simulink model "Mark60"  (Simulink 10.0)
settings: Solver=FixedStepAuto  StartTime=0.0  StopTime=4000  FixedStep=0.01  RelTol=1e-3  EnableMultiTasking=on
values from neighbouring files (symbols this model uses):
  A = 2.2    [constant（final）.m]
  c = 10800*0.9    (= 9720)    [constant（final）.m]
  C_D = 0.35    [constant（final）.m]
  C_e = 4.4    [constant（final）.m]
  C_t = 42    [constant（final）.m]
  Cb = interp1(SOC0,Cb0,SOC, 'spline')    [constant（final）.m]
  f = 0.018    [constant（final）.m]
  g = 9.8    [constant（final）.m]
  i_g = 2    [constant（final）.m]
  J_m = 0.25    [constant（final）.m]
  J_w = 4    [constant（final）.m]
  K_p = 4    [constant（final）.m]
  m = 1000    [constant（final）.m]
  Phi = 0.028    [constant（final）.m]
  r_w = 0.28    [constant（final）.m]
  Ra = 0.088    [constant（final）.m]
  Ro = interp1(SOC0,Ro0,SOC, 'spline')    [constant（final）.m]
  rou = 1.226    [constant（final）.m]
  Rp = interp1(SOC0,Rp0,SOC, 'spline')    [constant（final）.m]
  SOC = 0:0.0001:1    [constant（final）.m]
  T_i = 1    [constant（final）.m]
  tao = interp1(SOC0,tao0,SOC, 'spline')    [constant（final）.m]
  Uoc = UUoc*4.2/UUoc(10001)    [constant（final）.m]
  yita = 0.8    [constant（final）.m]
libraries: SignalEditorBlockLib x1
settings Model: Creator=TonyStark  LastModifiedBy=TonyStark
settings SolverCC: AutoInsertRateTranBlk=on
settings DataIOCC: LimitDataPoints=on  SignalLoggingSaveFormat=ModelDataLogs
settings OptimizationCC: ExpressionDepthLimit=2147483647
settings DebuggingCC: SolverPrmCheckMsg=warning  FcnCallInpInsideContextMsg=warning  StateNameClashWarn=warning
settings GRTTargetCC: GeneratePreprocessorConditionals=Disable all
settings ConfigComp: CovExternalEMLEnable=off

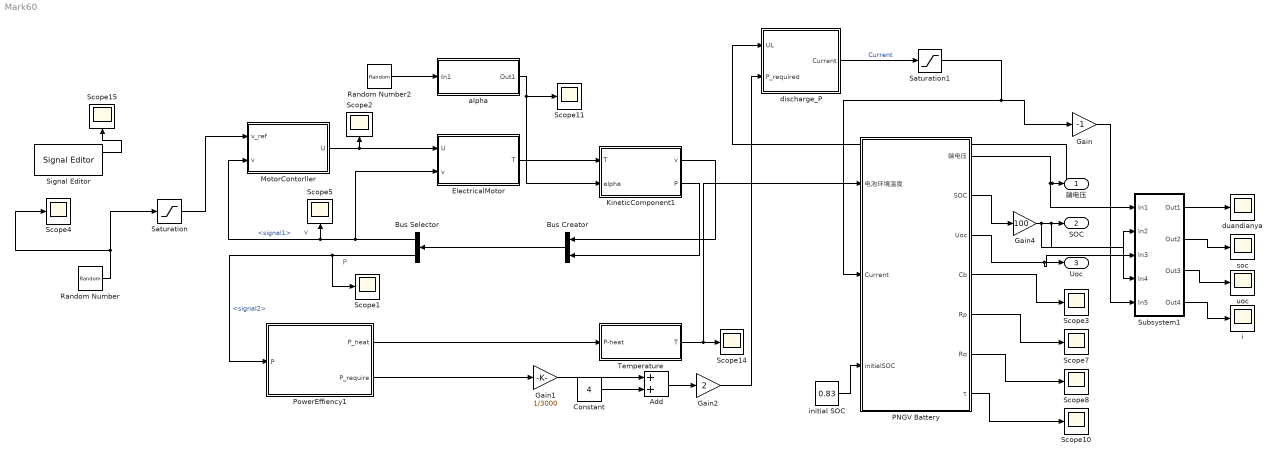
== system Mark60 ==
  note: v
  note: P
  Add : Sum
  Bus Creator : BusCreator  Inputs=2
  Bus Selector : BusSelector  OutputSignals=signal1,signal2
  Constant : Constant  Value=4
  ElectricalMotor : Subsystem
  Gain : Gain  Gain=-1
  Gain1 : Gain  Gain=1/3000
  Gain2 : Gain  Gain=2
  Gain4 : Gain  Gain=100
  KineticComponent1 : Subsystem
  MotorContorller : Subsystem
  PNGV Battery : Subsystem
  PowerEffiency1 : Subsystem
  Random Number : RandomNumber  Mean=13  Variance=2.5  Seed=2  SampleTime=0.01
  Random Number2 : RandomNumber  SampleTime=1
  Saturation : Saturate  UpperLimit=30  LowerLimit=0
  Saturation1 : Saturate  UpperLimit=100  LowerLimit=-100
  Scope{1..5,7..8,10..11,14..15} (11 alike) : Scope
  Signal Editor : SignalEditorBlockLib/Signal Editor  FileName=t1.mat  ActiveScenario=Scenario  ActiveSignal=Signal1  IsBus=off  OutputBusObjectStr=Bus: BusObject  SampleTime=0  Interpolate=off  ZeroCross=off  OutputAfterFinalValue=Setting to zero  Unit=inherit  PreserveSignalName=on
      settings: SourceProductName=Simulink
  Subsystem1 : Subsystem
  Temperature : Subsystem
  alpha : Subsystem
  discharge_P : Subsystem
  duandianya : Scope
  "i " : Scope
  initial SOC : Constant  Value=0.83
  "soc " : Scope
  "uoc " : Scope
  端电压 : Outport  VectorParamsAs1DForOutWhenUnconnected=off
  SOC : Outport  Port=2  VectorParamsAs1DForOutWhenUnconnected=off
  Uoc : Outport  Port=3  VectorParamsAs1DForOutWhenUnconnected=off
  wires:
  MotorContorller/1(U) -> ElectricalMotor/1(U), Scope2/1
  Bus Creator/1 -> Bus Selector/1
  Bus Selector/1 -> Scope5/1, MotorContorller/2(v), ElectricalMotor/2(v)  "<signal1>"
  KineticComponent1/1(v) -> Bus Creator/1
  KineticComponent1/2(P) -> Bus Creator/2
  ElectricalMotor/1(T) -> KineticComponent1/1(T)
  Bus Selector/2 -> Scope1/1, PowerEffiency1/1(P)  "<signal2>"
  PowerEffiency1/1(P_heat) -> Temperature/1(P-heat)
  Random Number2/1 -> alpha/1(In1)
  alpha/1(Out1) -> KineticComponent1/2(alpha), Scope11/1
  PNGV Battery/6(Ro) -> Scope8/1
  discharge_P/1(Current) -> Saturation1/1  "Current"
  Temperature/1(T) -> PNGV Battery/1(电池环境温度), Scope14/1
  Gain4/1 -> Subsystem1/4(In4), Subsystem1/2(In2), SOC/1
  initial SOC/1 -> PNGV Battery/3(initialSOC)
  PNGV Battery/4(Cb) -> Scope3/1
  PNGV Battery/7(τ) -> Scope10/1
  PNGV Battery/2(SOC) -> Gain4/1
  PNGV Battery/5(Rp) -> Scope7/1
  PowerEffiency1/2(P_require) -> Gain1/1
  Gain1/1 -> Add/1
  Add/1 -> Gain2/1
  Constant/1 -> Add/2
  Gain2/1 -> discharge_P/2(P_required)
  Random Number/1 -> Scope4/1, Saturation/1
  PNGV Battery/1(端电压) -> discharge_P/1(UL), 端电压/1, Subsystem1/1(In1)
  PNGV Battery/3(Uoc) -> Subsystem1/3(In3), Uoc/1
  Subsystem1/1(Out1) -> duandianya/1
  Subsystem1/2(Out2) -> "soc "/1
  Subsystem1/3(Out3) -> "uoc "/1
  Signal Editor/1 -> Scope15/1
  Subsystem1/4(Out4) -> "i "/1
  Gain/1 -> Subsystem1/5(In5)
  Saturation1/1 -> PNGV Battery/2(Current), Gain/1
  Saturation/1 -> MotorContorller/1(v_ref)

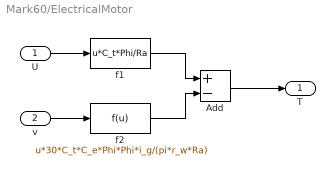
== system Mark60/ElectricalMotor ==
  U : Inport
  v : Inport  Port=2
  Add : Sum  Inputs=+-
  f1 : Fcn  Expr=u*C_t*Phi/Ra
  f2 : Fcn  Expr=u*30*C_t*C_e*Phi*Phi*i_g/(pi*r_w*Ra)
  T : Outport  VectorParamsAs1DForOutWhenUnconnected=off
  wires:
  U/1 -> f1/1
  v/1 -> f2/1
  f1/1 -> Add/1
  f2/1 -> Add/2
  Add/1 -> T/1

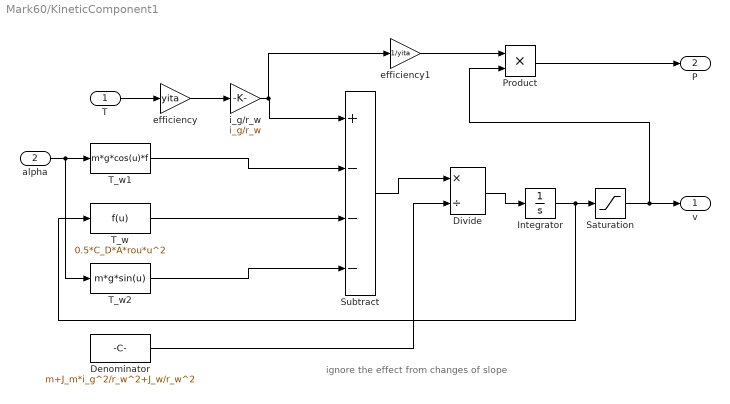
== system Mark60/KineticComponent1 ==
  note: ignore the effect from changes of slope
  T : Inport
  alpha : Inport  Port=2
  Denominator : Constant  Value=m+J_m*i_g^2/r_w^2+J_w/r_w^2
  Divide : Product  Inputs=*/
  Integrator : Integrator
  Product : Product  RndMeth=Zero
  Saturation : Saturate  UpperLimit=inf  LowerLimit=0
  Subtract : Sum  Inputs=+---
  T_w : Fcn  Expr=0.5*C_D*A*rou*u^2
  T_w1 : Fcn  Expr=m*g*cos(u)*f
  T_w2 : Fcn  Expr=m*g*sin(u)
  efficiency : Gain  Gain=yita
  efficiency1 : Gain  Gain=1/yita
  i_g/r_w : Gain  Gain=i_g/r_w
  v : Outport  VectorParamsAs1DForOutWhenUnconnected=off
  P : Outport  Port=2  VectorParamsAs1DForOutWhenUnconnected=off
  wires:
  efficiency/1 -> i_g/r_w/1
  i_g/r_w/1 -> Subtract/1, efficiency1/1
  T_w/1 -> Subtract/3
  Subtract/1 -> Divide/1
  Divide/1 -> Integrator/1
  Integrator/1 -> Saturation/1, T_w/1
  Denominator/1 -> Divide/2
  Product/1 -> P/1
  Saturation/1 -> v/1, Product/2
  T/1 -> efficiency/1
  efficiency1/1 -> Product/1
  alpha/1 -> T_w1/1, T_w2/1
  T_w2/1 -> Subtract/4
  T_w1/1 -> Subtract/2

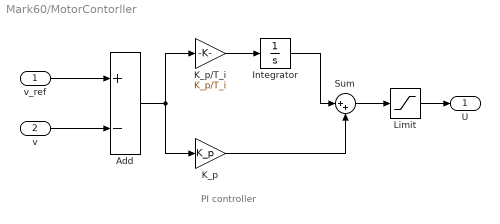
== system Mark60/MotorContorller ==
  note: PI controller
  v_ref : Inport
  v : Inport  Port=2
  Add : Sum  Inputs=+-
  Integrator : Integrator
  K_p : Gain  Gain=K_p
  K_p/T_i : Gain  Gain=K_p/T_i
  Limit : Saturate  UpperLimit=inf  LowerLimit=-inf
  Sum : Sum  Inputs=|++
  U : Outport  VectorParamsAs1DForOutWhenUnconnected=off
  wires:
  v_ref/1 -> Add/1
  v/1 -> Add/2
  Add/1 -> K_p/1, K_p/T_i/1
  K_p/T_i/1 -> Integrator/1
  Limit/1 -> U/1
  Sum/1 -> Limit/1
  K_p/1 -> Sum/2
  Integrator/1 -> Sum/1

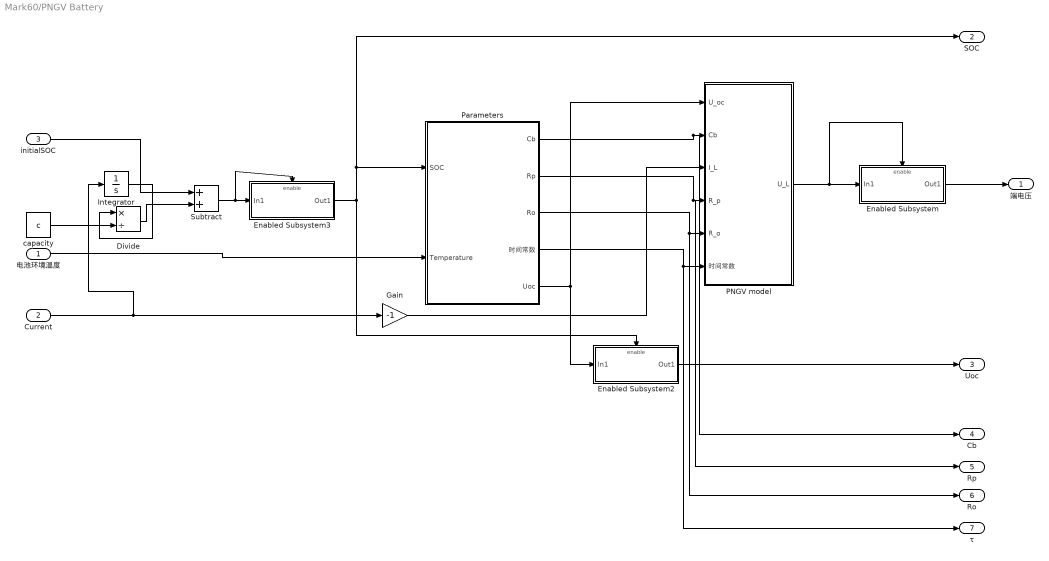
== system Mark60/PNGV Battery ==
  电池环境温度 : Inport
  Current : Inport  Port=2
  initialSOC : Inport  Port=3
  Divide : Product  Inputs=*/
  Enabled Subsystem : Subsystem  TreatAsAtomicUnit=on
  Enabled Subsystem2 : Subsystem  TreatAsAtomicUnit=on
  Enabled Subsystem3 : Subsystem  TreatAsAtomicUnit=on
  Gain : Gain  Gain=-1
  Integrator : Integrator
  PNGV model : Subsystem
  Parameters : Subsystem  TreatAsAtomicUnit=on
  Subtract : Sum
  capacity : Constant  Value=c
  端电压 : Outport  VectorParamsAs1DForOutWhenUnconnected=off
  SOC : Outport  Port=2  VectorParamsAs1DForOutWhenUnconnected=off
  Uoc : Outport  Port=3  VectorParamsAs1DForOutWhenUnconnected=off
  Cb : Outport  Port=4  VectorParamsAs1DForOutWhenUnconnected=off
  Rp : Outport  Port=5  VectorParamsAs1DForOutWhenUnconnected=off
  Ro : Outport  Port=6  VectorParamsAs1DForOutWhenUnconnected=off
  τ : Outport  Port=7  VectorParamsAs1DForOutWhenUnconnected=off
  wires:
  Current/1 -> Integrator/1, Gain/1
  电池环境温度/1 -> Parameters/2(Temperature)
  Enabled Subsystem2/1(Out1) -> Uoc/1
  Parameters/5(Uoc) -> PNGV model/1(U_oc), Enabled Subsystem2/1(In1)
  Subtract/1 -> Enabled Subsystem3/1(In1), Enabled Subsystem3/Enable
  Enabled Subsystem/1(Out1) -> 端电压/1
  Enabled Subsystem3/1(Out1) -> SOC/1, Parameters/1(SOC), Enabled Subsystem2/Enable
  Parameters/3(Ro) -> PNGV model/5(R_o), Ro/1
  capacity/1 -> Divide/2
  Parameters/4(时间常数) -> τ/1, PNGV model/6(时间常数)
  Integrator/1 -> Divide/1
  Parameters/1(Cb) -> Cb/1, PNGV model/2(Cb)
  PNGV model/1(U_L) -> Enabled Subsystem/Enable, Enabled Subsystem/1(In1)
  Divide/1 -> Subtract/2
  Parameters/2(Rp) -> Rp/1, PNGV model/4(R_p)
  Gain/1 -> PNGV model/3(I_L)
  initialSOC/1 -> Subtract/1

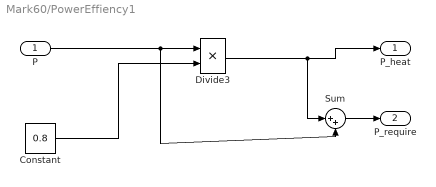
== system Mark60/PowerEffiency1 ==
  P : Inport
  Constant : Constant  Value=0.8
  Divide3 : Product  Inputs=**
  Sum : Sum  Inputs=|++
  P_heat : Outport  VectorParamsAs1DForOutWhenUnconnected=off
  P_require : Outport  Port=2  VectorParamsAs1DForOutWhenUnconnected=off
  wires:
  Sum/1 -> P_require/1
  Constant/1 -> Divide3/2
  Divide3/1 -> Sum/1, P_heat/1
  P/1 -> Divide3/1, Sum/2

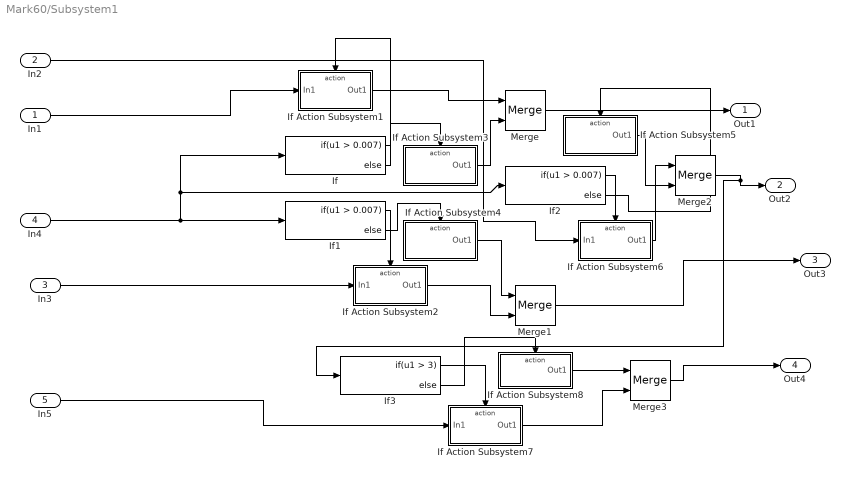
== system Mark60/Subsystem1 ==
  In1 : Inport
  In2 : Inport  Port=2
  In3 : Inport  Port=3
  In4 : Inport  Port=4
  In5 : Inport  Port=5
  If : If  IfExpression=u1 > 0.007
  If Action Subsystem1 : Subsystem  TreatAsAtomicUnit=on
  If Action Subsystem2 : Subsystem  TreatAsAtomicUnit=on
  If Action Subsystem3 : Subsystem  TreatAsAtomicUnit=on
  If Action Subsystem4 : Subsystem  TreatAsAtomicUnit=on
  If Action Subsystem5 : Subsystem  TreatAsAtomicUnit=on
  If Action Subsystem6 : Subsystem  TreatAsAtomicUnit=on
  If Action Subsystem7 : Subsystem  TreatAsAtomicUnit=on
  If Action Subsystem8 : Subsystem  TreatAsAtomicUnit=on
  If1 : If  IfExpression=u1 > 0.007
  If2 : If  IfExpression=u1 > 0.007
  If3 : If  IfExpression=u1 > 3
  Merge{,1..3} (4 alike) : Merge
  Out1 : Outport
  Out2 : Outport  Port=2
  Out3 : Outport  Port=3
  Out4 : Outport  Port=4
  wires:
  If2/2 -> If Action Subsystem5/Action
  If Action Subsystem3/1(Out1) -> Merge/2
  If1/1 -> If Action Subsystem2/Action
  If Action Subsystem2/1(Out1) -> Merge1/2
  If/2 -> If Action Subsystem3/Action
  If/1 -> If Action Subsystem1/Action
  If Action Subsystem4/1(Out1) -> Merge1/1
  If2/1 -> If Action Subsystem6/Action
  If Action Subsystem6/1(Out1) -> Merge2/1
  If1/2 -> If Action Subsystem4/Action
  If Action Subsystem1/1(Out1) -> Merge/1
  If Action Subsystem5/1(Out1) -> Merge2/2
  In4/1 -> If2/1, If/1, If1/1
  In2/1 -> If Action Subsystem6/1(In1)
  Merge1/1 -> Out3/1
  In1/1 -> If Action Subsystem1/1(In1)
  Merge/1 -> Out1/1
  If3/1 -> If Action Subsystem7/Action
  Merge3/1 -> Out4/1
  If Action Subsystem7/1(Out1) -> Merge3/2
  If Action Subsystem8/1(Out1) -> Merge3/1
  If3/2 -> If Action Subsystem8/Action
  In3/1 -> If Action Subsystem2/1(In1)
  In5/1 -> If Action Subsystem7/1(In1)
  Merge2/1 -> If3/1, Out2/1

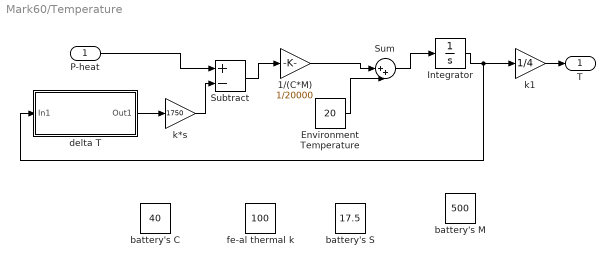
== system Mark60/Temperature ==
  P-heat : Inport
  1/(C*M) : Gain  Gain=1/20000
  Environment Temperature : Constant  Value=20
  Integrator : Integrator
  Subtract : Sum  Inputs=+-
  Sum : Sum  Inputs=|++
  battery's C : Constant  Value=40
  battery's M : Constant  Value=500
  battery's S : Constant  Value=17.5
  delta T : Subsystem
  fe-al thermal k : Constant  Value=100
  k*s : Gain  Gain=1750
  k1 : Gain  Gain=1/4
  T : Outport  VectorParamsAs1DForOutWhenUnconnected=off
  wires:
  delta T/1(Out1) -> k*s/1
  k*s/1 -> Subtract/2
  1/(C*M)/1 -> Sum/1
  P-heat/1 -> Subtract/1
  Environment Temperature/1 -> Sum/2
  Sum/1 -> Integrator/1
  Integrator/1 -> delta T/1(In1), k1/1
  Subtract/1 -> 1/(C*M)/1
  k1/1 -> T/1

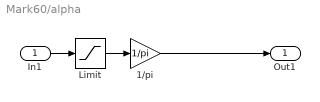
== system Mark60/alpha ==
  In1 : Inport
  1/pi : Gain  Gain=1/pi
  Limit : Saturate  UpperLimit=pi/4  LowerLimit=-pi/4
  Out1 : Outport  VectorParamsAs1DForOutWhenUnconnected=off
  wires:
  In1/1 -> Limit/1
  1/pi/1 -> Out1/1
  Limit/1 -> 1/pi/1

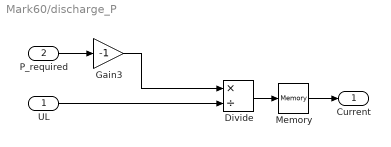
== system Mark60/discharge_P ==
  UL : Inport
  P_required : Inport  Port=2
  Divide : Product  Inputs=*/
  Gain3 : Gain  Gain=-1
  Memory : Memory  InitialCondition=1  InheritSampleTime=on
  Current : Outport  VectorParamsAs1DForOutWhenUnconnected=off
  wires:
  P_required/1 -> Gain3/1
  UL/1 -> Divide/2
  Divide/1 -> Memory/1
  Memory/1 -> Current/1
  Gain3/1 -> Divide/1

== system Mark60/PNGV Battery/Enabled Subsystem ==
  In1 : Inport
  Enable : EnablePort
  Out1 : Outport  VectorParamsAs1DForOutWhenUnconnected=off
  wires:
  In1/1 -> Out1/1

== system Mark60/PNGV Battery/Enabled Subsystem2 ==
  In1 : Inport
  Enable : EnablePort
  Out1 : Outport  VectorParamsAs1DForOutWhenUnconnected=off
  wires:
  In1/1 -> Out1/1

== system Mark60/PNGV Battery/Enabled Subsystem3 ==
  In1 : Inport
  Enable : EnablePort
  Out1 : Outport  VectorParamsAs1DForOutWhenUnconnected=off
  wires:
  In1/1 -> Out1/1

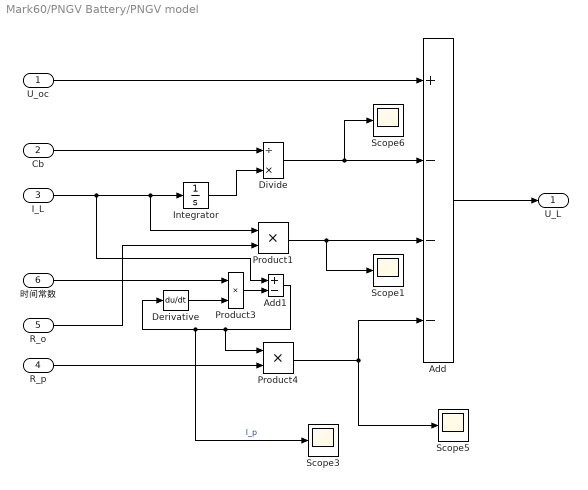
== system Mark60/PNGV Battery/PNGV model ==
  U_oc : Inport
  Cb : Inport  Port=2
  I_L : Inport  Port=3
  R_p : Inport  Port=4
  R_o : Inport  Port=5
  时间常数 : Inport  Port=6
  Add : Sum  Inputs=+---
  Add1 : Sum  Inputs=+-
  Derivative : Derivative
  Divide : Product  Inputs=/*
  Integrator : Integrator
  Product1 : Product
  Product3 : Product
  Product4 : Product
  Scope{1,3,5..6} (4 alike) : Scope
  U_L : Outport  VectorParamsAs1DForOutWhenUnconnected=off
  wires:
  Add/1 -> U_L/1
  Cb/1 -> Divide/1
  Integrator/1 -> Divide/2
  I_L/1 -> Add1/1, Product1/1, Integrator/1
  Divide/1 -> Scope6/1, Add/2
  Product1/1 -> Scope1/1, Add/3
  R_o/1 -> Product1/2
  时间常数/1 -> Product3/1
  Product3/1 -> Add1/2
  Derivative/1 -> Product3/2
  Add1/1 -> Product4/1, Scope3/1, Derivative/1  "I_p"
  R_p/1 -> Product4/2
  Product4/1 -> Scope5/1, Add/4
  U_oc/1 -> Add/1

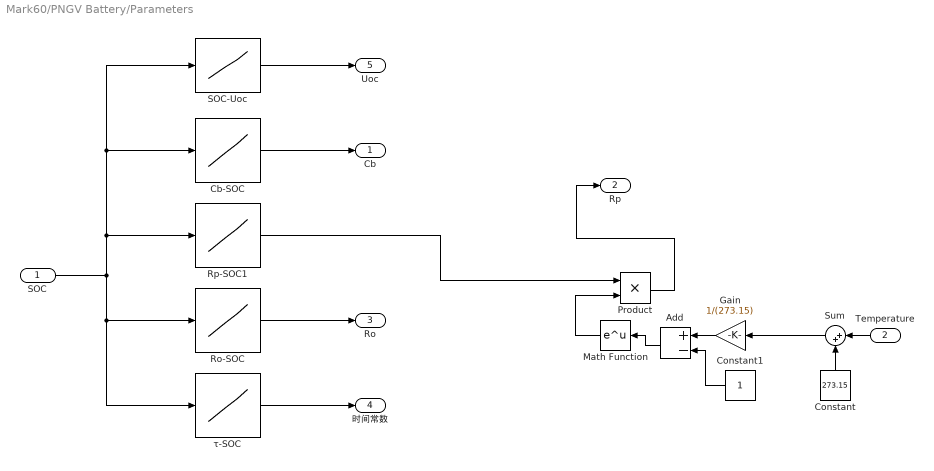
== system Mark60/PNGV Battery/Parameters ==
  SOC : Inport
  Temperature : Inport  Port=2
  Add : Sum  Inputs=+-
  Cb-SOC : Lookup_n-D  NumberOfTableDimensions=1  BreakpointsForDimension1=SOC  Table=Cb  InterpMethod=Linear Lagrange  UseLastTableValue=on  InternalRulePriority=Speed  RndMeth=Simplest  InputSameDT=on
  Constant : Constant  Value=273.15
  Constant1 : Constant
  Gain : Gain  Gain=1/(273.15)
  Math Function : Math  SaturateOnIntegerOverflow=on
  Product : Product
  Ro-SOC : Lookup_n-D  NumberOfTableDimensions=1  BreakpointsForDimension1=SOC  Table=Ro  InterpMethod=Linear Lagrange  UseLastTableValue=on  InternalRulePriority=Speed  RndMeth=Simplest  InputSameDT=on
  Rp-SOC1 : Lookup_n-D  NumberOfTableDimensions=1  BreakpointsForDimension1=SOC  Table=Rp  InterpMethod=Linear Lagrange  UseLastTableValue=on  InternalRulePriority=Speed  RndMeth=Simplest  InputSameDT=on
  SOC-Uoc : Lookup_n-D  NumberOfTableDimensions=1  BreakpointsForDimension1=SOC  Table=Uoc  InterpMethod=Linear Lagrange  InternalRulePriority=Speed  RndMeth=Simplest  InputSameDT=on
  Sum : Sum  Inputs=|++
  τ-SOC : Lookup_n-D  NumberOfTableDimensions=1  BreakpointsForDimension1=SOC  Table=tao  InterpMethod=Linear Lagrange  UseLastTableValue=on  InternalRulePriority=Speed  RndMeth=Simplest  InputSameDT=on
  Cb : Outport  VectorParamsAs1DForOutWhenUnconnected=off
  Rp : Outport  Port=2  VectorParamsAs1DForOutWhenUnconnected=off
  Ro : Outport  Port=3  VectorParamsAs1DForOutWhenUnconnected=off
  时间常数 : Outport  Port=4  VectorParamsAs1DForOutWhenUnconnected=off
  Uoc : Outport  Port=5  VectorParamsAs1DForOutWhenUnconnected=off
  wires:
  SOC/1 -> SOC-Uoc/1, Cb-SOC/1, Rp-SOC1/1, τ-SOC/1, Ro-SOC/1
  Cb-SOC/1 -> Cb/1
  Ro-SOC/1 -> Ro/1
  τ-SOC/1 -> 时间常数/1
  SOC-Uoc/1 -> Uoc/1
  Sum/1 -> Gain/1
  Math Function/1 -> Product/2
  Constant/1 -> Sum/2
  Temperature/1 -> Sum/1
  Rp-SOC1/1 -> Product/1
  Product/1 -> Rp/1
  Gain/1 -> Add/1
  Add/1 -> Math Function/1
  Constant1/1 -> Add/2

== system Mark60/Subsystem1/If Action Subsystem1 ==
  In1 : Inport
  Action Port : ActionPort  ActionPortLabel=if(u1 > 0.007)
  Out1 : Outport
  wires:
  In1/1 -> Out1/1

== system Mark60/Subsystem1/If Action Subsystem2 ==
  In1 : Inport
  Action Port : ActionPort  ActionPortLabel=if(u1 > 0.007)
  Out1 : Outport
  wires:
  In1/1 -> Out1/1

== system Mark60/Subsystem1/If Action Subsystem3 ==
  Action Port : ActionPort  ActionPortLabel=else
  Constant : Constant  Value=0
  Out1 : Outport
  wires:
  Constant/1 -> Out1/1

== system Mark60/Subsystem1/If Action Subsystem4 ==
  Action Port : ActionPort  ActionPortLabel=else
  Constant : Constant  Value=0
  Out1 : Outport
  wires:
  Constant/1 -> Out1/1

== system Mark60/Subsystem1/If Action Subsystem5 ==
  Action Port : ActionPort  ActionPortLabel=else
  Constant : Constant  Value=0
  Out1 : Outport
  wires:
  Constant/1 -> Out1/1

== system Mark60/Subsystem1/If Action Subsystem6 ==
  In1 : Inport
  Action Port : ActionPort  ActionPortLabel=if(u1 > 0.007)
  Out1 : Outport
  wires:
  In1/1 -> Out1/1

== system Mark60/Subsystem1/If Action Subsystem7 ==
  In1 : Inport
  Action Port : ActionPort  ActionPortLabel=if(u1 > 3)
  Out1 : Outport
  wires:
  In1/1 -> Out1/1

== system Mark60/Subsystem1/If Action Subsystem8 ==
  Action Port : ActionPort  ActionPortLabel=else
  Constant : Constant  Value=0
  Out1 : Outport
  wires:
  Constant/1 -> Out1/1

== system Mark60/Temperature/delta T ==
  In1 : Inport
  Add : Sum  Inputs=+-
  Environment Temperature : Constant  Value=20
  Out1 : Outport  VectorParamsAs1DForOutWhenUnconnected=off
  wires:
  In1/1 -> Add/1
  Add/1 -> Out1/1
  Environment Temperature/1 -> Add/2
